simulink model "b"  (R2012b)
settings: Solver=ode45  StartTime=data(1,1)  StopTime=data(end,1)  RelTol=1e-3
PreLoadFcn:
  | add_data;
settings Model: Creator=ZhouHaoyu  LastModifiedBy=ZhouHaoyu
settings DataIOCC: ExternalInput=[data(:,1), data(:,2)]  LoadExternalInput=on

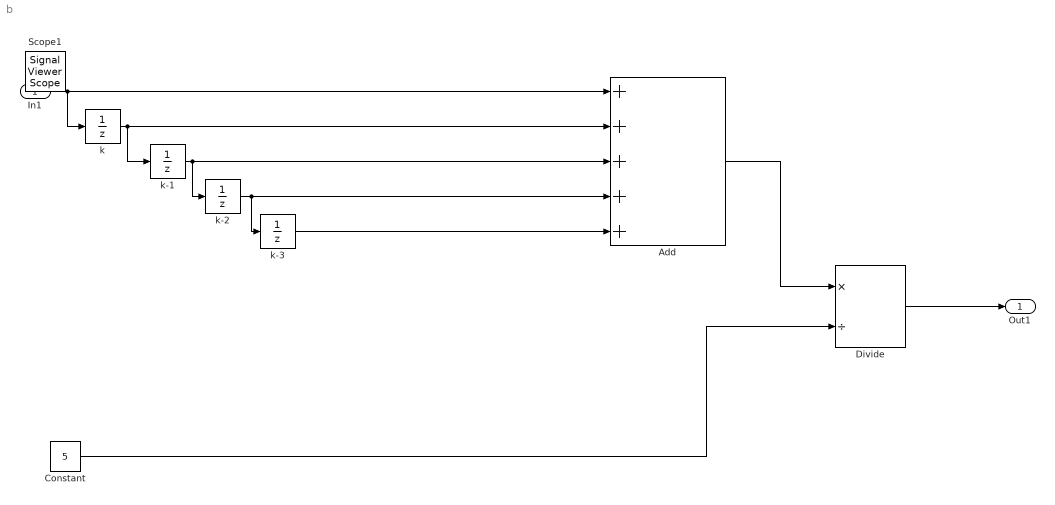
== system b ==
  In1 : Inport
  Add : Sum  Inputs=+++++
  Constant : Constant  Value=5
  Divide : Product  Inputs=*/
  k : UnitDelay  SampleTime=-1
  k-1 : UnitDelay  SampleTime=-1
  k-2 : UnitDelay  SampleTime=-1
  k-3 : UnitDelay  SampleTime=-1
  Out1 : Outport
  Scope1 : SignalViewerScope  IOType=viewer  RefreshTime=0.035000
  wires:
  In1/1 -> Add/1, k/1
  k/1 -> k-1/1, Add/2
  k-1/1 -> k-2/1, Add/3
  k-2/1 -> k-3/1, Add/4
  Add/1 -> Divide/1
  Constant/1 -> Divide/2
  Divide/1 -> Out1/1
  k-3/1 -> Add/5
